simulink model "Ex9_9model"  (R2013a)
settings: Solver=ode45  StartTime=0.0  StopTime=10.0  RelTol=1e-3
settings Model: Creator=JLS  LastModifiedBy=John
settings DataIOCC: SignalLoggingSaveFormat=ModelDataLogs
settings OptimizationCC: ExpressionDepthLimit=2147483647
settings DebuggingCC: FcnCallInpInsideContextMsg=UseLocalSettings
settings GRTTargetCC: CombineOutputUpdateFcns=off  GRTInterface=on

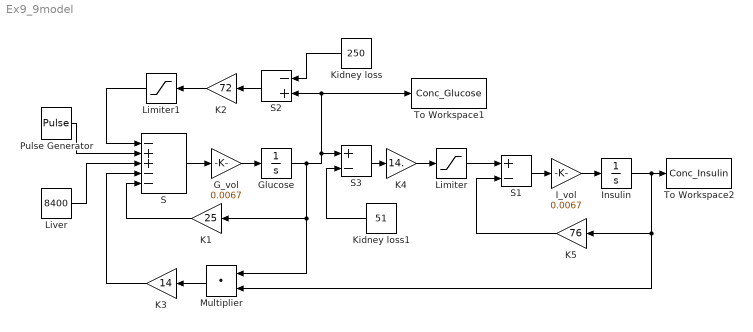
== system Ex9_9model ==
  G_vol : Gain  Gain=0.0067
  Glucose : Integrator  InitialCondition=81
  I_vol : Gain  Gain=0.0067
  Insulin : Integrator  InitialCondition=5.66
  K1 : Gain  Gain=25
  "K2 " : Gain  Gain=72
  K3 : Gain  Gain=14
  K4 : Gain  Gain=14.
  K5 : Gain  Gain=76
  Kidney loss : Constant  Value=250
  Kidney loss1 : Constant  Value=51
  Limiter : Saturate  UpperLimit=10000  LowerLimit=0
  Limiter1 : Saturate  UpperLimit=10000  LowerLimit=0
  Liver : Constant  Value=8400
  Multiplier : DotProduct  InputSameDT=on  OutDataTypeStr=Inherit: Inherit via internal rule
  Pulse Generator : DiscretePulseGenerator  PulseType=Time based  Amplitude=80000  Period=20  PulseWidth=2.5  PhaseDelay=1
  S : Sum  Inputs=-++--
  S1 : Sum  Inputs=+-
  S2 : Sum  Inputs=-+
  S3 : Sum  Inputs=+-
  To Workspace1 : ToWorkspace  VariableName=Conc_Glucose  SampleTime=-1
  To Workspace2 : ToWorkspace  VariableName=Conc_Insulin  SampleTime=-1
  wires:
  K4/1 -> Limiter/1
  Limiter/1 -> S1/1
  Insulin/1 -> To Workspace2/1, K5/1, Multiplier/2
  K5/1 -> S1/2
  Glucose/1 -> K1/1, Multiplier/1, S3/1, To Workspace1/1, S2/2
  K1/1 -> S/5
  Pulse Generator/1 -> S/2
  Liver/1 -> S/3
  K3/1 -> S/4
  Multiplier/1 -> K3/1
  "K2 "/1 -> Limiter1/1
  Limiter1/1 -> S/1
  G_vol/1 -> Glucose/1
  S/1 -> G_vol/1
  I_vol/1 -> Insulin/1
  S1/1 -> I_vol/1
  S2/1 -> "K2 "/1
  Kidney loss/1 -> S2/1
  S3/1 -> K4/1
  Kidney loss1/1 -> S3/2
